simulink model "LQR_simulink"  (R2023a)
settings: Solver=VariableStepAuto  StartTime=0.0  StopTime=10.0  RelTol=1e-3
undefined symbols (not defined in the file): A_mat, B_mat, C_mat, K
settings Model: Creator=Shehab Abdo  LastModifiedBy=Shehab Abdo

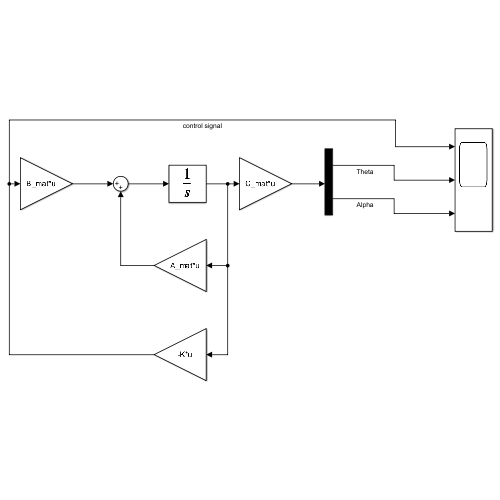
[thumbnail: Simulink's stored preview of the top-level diagram]
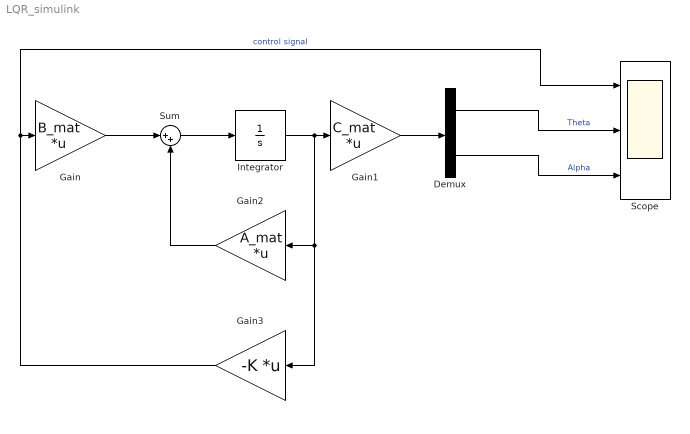
== system LQR_simulink ==
  Demux : Demux  Outputs=2
  Gain : Gain  Gain=B_mat  Multiplication=Matrix(K*u)
  Gain1 : Gain  Gain=C_mat  Multiplication=Matrix(K*u)
  Gain2 : Gain  Gain=A_mat  Multiplication=Matrix(K*u)
  Gain3 : Gain  Gain=-K  Multiplication=Matrix(K*u)
  Integrator : Integrator  InitialCondition=[0.9 0.47 0 0]
  Scope : Scope  NumInputPorts=3
  Sum : Sum  Inputs=|++
  wires:
  Gain/1 -> Sum/1
  Sum/1 -> Integrator/1
  Integrator/1 -> Gain2/1, Gain3/1, Gain1/1
  Gain1/1 -> Demux/1
  Gain2/1 -> Sum/2
  Gain3/1 -> Scope/1, Gain/1  "control signal"
  Demux/2 -> Scope/3  "Alpha"
  Demux/1 -> Scope/2  "Theta"
